simulink model "dynamics_working_version_02_12"  (R2019a)
settings: Solver=FixedStepAuto  StartTime=0.0  StopTime=10.0  FixedStep=3.90625e-3  RelTol=1e-3
values from neighbouring files (symbols this model uses):
  b = 0.033    [set_params.m]
  g = 9.81    [set_params.m]
  I_CF_1 = [16.823890  -1.224320  -0.716891 ... (first row only)    [set_params.m]
  I_CF_1_inv = inv(I_CF_1)    [set_params.m]
  I_rzz = 9.3e-6    (= 9.3e-06)    [set_params.m]
  k_f = 1.6e-4    (= 0.00016)    [set_params.m]
  k_m = 1e-8    (= 1e-08)    [set_params.m]
  kx = 10.25e-4    (= 0.001025)    [set_params.m]
  ky = 10.25e-4    (= 0.001025)    [set_params.m]
  kz = 7.553e-4    (= 0.0007553)    [set_params.m]
  l = 0.033    [set_params.m]
  m_CF = 0.028    [set_params.m]
  omega_n = 50    [set_params.m]
  T = 1/15    (= 0.0666666666667)    [inner_pd.m]    (also in inner_pd_cs.m; outer_pd.m; outer_pd_cs.m; set_params.m)
  zeta = 0.55    [set_params.m]
libraries: sharedutil x2, simulink x1
settings Model: Creator=evgheniivolodscoi  LastModifiedBy=evgheniivolodscoi

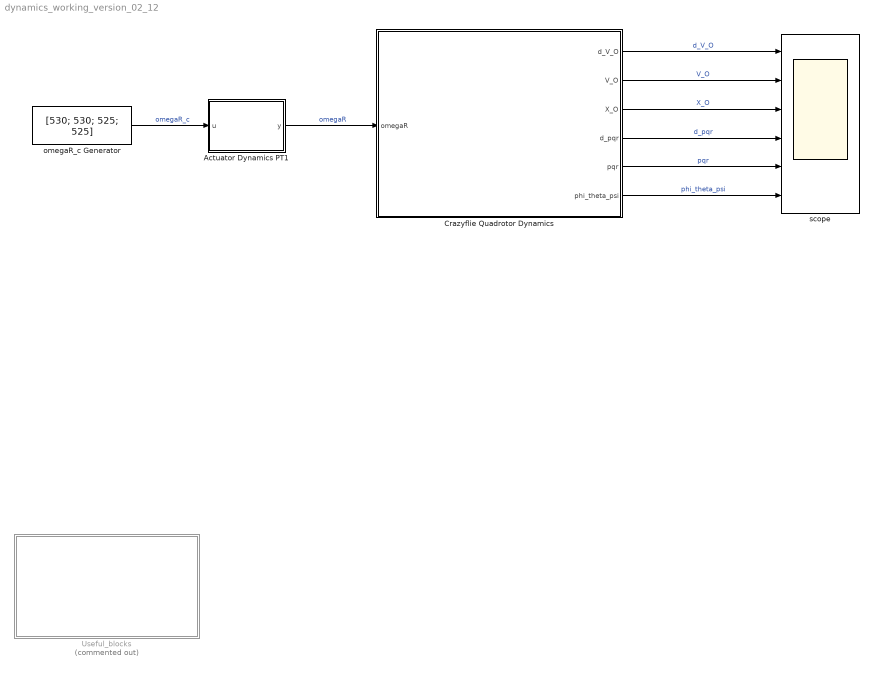
== system dynamics_working_version_02_12 ==
  Actuator Dynamics PT1 : Subsystem
  Crazyflie Quadrotor Dynamics : Subsystem
  "Useful_blocks " : Subsystem  Commented=on
  "omegaR_c Generator " : Constant  Value=[530; 530; 525; 525]
  scope : Scope  NumInputPorts=6
  wires:
  Crazyflie Quadrotor Dynamics/6(phi_theta_psi) -> scope/6  "phi_theta_psi"
  Actuator Dynamics PT1/1(y) -> Crazyflie Quadrotor Dynamics/1(omegaR)  "omegaR"
  Crazyflie Quadrotor Dynamics/4(d_pqr) -> scope/4  "d_pqr"
  Crazyflie Quadrotor Dynamics/3(X_O) -> scope/3  "X_O"
  Crazyflie Quadrotor Dynamics/2(V_O) -> scope/2  "V_O"
  Crazyflie Quadrotor Dynamics/1(d_V_O) -> scope/1  "d_V_O"
  "omegaR_c Generator "/1 -> Actuator Dynamics PT1/1(u)  "omegaR_c"
  Crazyflie Quadrotor Dynamics/5(pqr) -> scope/5  "pqr"

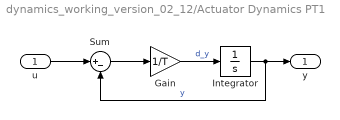
== system dynamics_working_version_02_12/Actuator Dynamics PT1 ==
  u : Inport
  Gain : Gain  Gain=1/T
  Integrator : Integrator
  Sum : Sum  Inputs=|+-
  y : Outport
  wires:
  Integrator/1 -> Sum/2, y/1  "y"
  u/1 -> Sum/1
  Gain/1 -> Integrator/1  "d_y"
  Sum/1 -> Gain/1

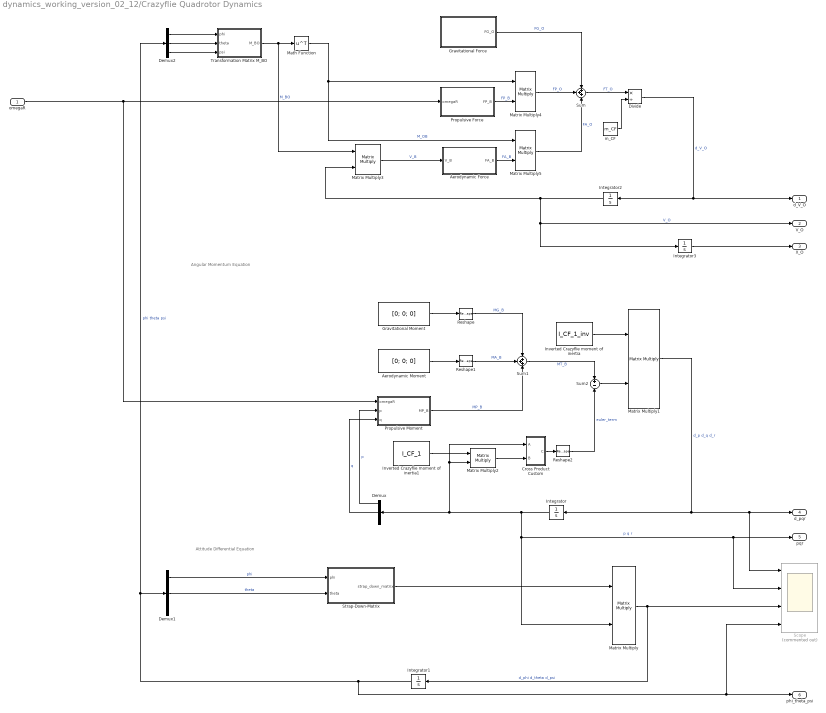
== system dynamics_working_version_02_12/Crazyflie Quadrotor Dynamics ==
  note: Angular Momentum Equation
  note: Attitude Differential Equation
  omegaR : Inport
  Aerodynamic Force : Subsystem
  Aerodynamic Moment : Constant  Value=[0; 0; 0]
  Cross Product Custom : Subsystem
  Demux : Demux  Outputs=3
  Demux1 : Demux  Outputs=3
  Demux2 : Demux  Outputs=3
  Divide : Product  Inputs=*/
  "Gravitational Force " : Subsystem
  Gravitational Moment : Constant  Value=[0; 0; 0]
  Integrator{,1..3} (4 alike) : Integrator  InitialCondition=[0; 0; 0]
  Inverted Crazyflie moment of inertia : Constant  Value=I_CF_1_inv
  Inverted Crazyflie moment of inertia1 : Constant  Value=I_CF_1
  Math Function : Math  Operator=transpose  SaturateOnIntegerOverflow=on
  Matrix Multiply{,1..5} (6 alike) : Product  Multiplication=Matrix(*)
  Propulsive Force : Subsystem
  Propulsive Moment : Subsystem
  Reshape : Reshape  OutputDimensionality=Column vector (2-D)
  Reshape1 : Reshape  OutputDimensionality=Column vector (2-D)
  Reshape2 : Reshape  OutputDimensionality=Column vector (2-D)
  Scope : Scope  Commented=on  NumInputPorts=4
  Strap-Down-Matrix : Subsystem
  Sum : Sum  Inputs=+++
  Sum1 : Sum  Inputs=+++
  Sum2 : Sum  Inputs=+-
  Transformation Matrix M_BO : Subsystem
  m_CF : Constant  Value=m_CF
  d_V_O : Outport
  V_O : Outport  Port=2
  X_O : Outport  Port=3
  d_pqr : Outport  Port=4
  pqr : Outport  Port=5
  phi_theta_psi : Outport  Port=6
  wires:
  Aerodynamic Moment/1 -> Reshape1/1
  Matrix Multiply1/1 -> Integrator/1, Scope/1, d_pqr/1  "d_p d_q d_r"
  Demux1/2 -> Strap-Down-Matrix/2(theta)  "theta"
  Inverted Crazyflie moment of inertia/1 -> Matrix Multiply1/1
  Integrator1/1 -> Demux2/1, Demux1/1, Scope/4, phi_theta_psi/1  "phi theta psi"
  Demux/1 -> Propulsive Moment/2(p)  "p"
  Integrator/1 -> Demux/1, Cross Product Custom/1(A), Matrix Multiply2/2, Matrix Multiply/2, Scope/2, pqr/1  "p q r"
  Propulsive Force/1(FP_B) -> Matrix Multiply4/2  "FP_B"
  "Gravitational Force "/1(FG_O) -> Sum/1  "FG_O"
  Matrix Multiply4/1 -> Sum/2  "FP_O"
  Propulsive Moment/1(MP_B) -> Sum1/3  "MP_B"
  Sum/1 -> Divide/1  "FT_O"
  Demux2/2 -> Transformation Matrix M_BO/2(theta)
  m_CF/1 -> Divide/2
  Gravitational Moment/1 -> Reshape/1
  Transformation Matrix M_BO/1(M_BO) -> Matrix Multiply3/1, Math Function/1  "M_BO"
  Aerodynamic Force/1(FA_B) -> Matrix Multiply5/2  "FA_B"
  Matrix Multiply2/1 -> Cross Product Custom/2(B)
  Cross Product Custom/1(C) -> Reshape2/1
  Matrix Multiply/1 -> Integrator1/1, Scope/3  "d_phi d_theta d_psi"
  Matrix Multiply3/1 -> Aerodynamic Force/1(V_B)  "V_B"
  Demux2/1 -> Transformation Matrix M_BO/1(phi)
  Math Function/1 -> Matrix Multiply4/1, Matrix Multiply5/1  "M_OB"
  Matrix Multiply5/1 -> Sum/3  "FA_O"
  Strap-Down-Matrix/1(strap_down_matrix) -> Matrix Multiply/1
  Demux2/3 -> Transformation Matrix M_BO/3(psi)
  Demux1/1 -> Strap-Down-Matrix/1(phi)  "phi"
  Sum1/1 -> Sum2/1  "MT_B"
  Demux/2 -> Propulsive Moment/3(q)  "q"
  Reshape/1 -> Sum1/1  "MG_B"
  Reshape1/1 -> Sum1/2  "MA_B"
  Reshape2/1 -> Sum2/2  "euler_term"
  omegaR/1 -> Propulsive Moment/1(omegaR), Propulsive Force/1(omegaR)
  Divide/1 -> d_V_O/1, Integrator2/1  "d_V_O"
  Integrator2/1 -> Integrator3/1, V_O/1, Matrix Multiply3/2  "V_O"
  Integrator3/1 -> X_O/1
  Sum2/1 -> Matrix Multiply1/2
  Inverted Crazyflie moment of inertia1/1 -> Matrix Multiply2/1

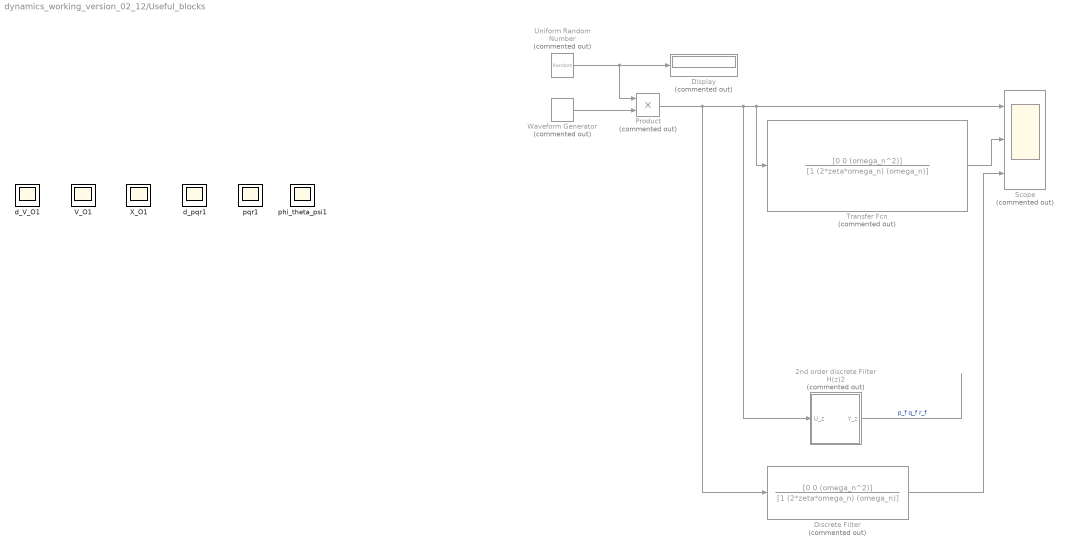
== system dynamics_working_version_02_12/Useful_blocks  ==
  2nd order discrete Filter H(z)2 : Subsystem  Commented=on
  Discrete Filter : DiscreteFilter  Commented=on  Numerator=[0 0 (omega_n^2)]  Denominator=[1 (2*zeta*omega_n) (omega_n)]
  Display : Display  Commented=on
  Product : Product  Commented=on
  Scope : Scope  Commented=on  NumInputPorts=3
  Transfer Fcn : TransferFcn  Commented=on  Numerator=[0 0 (omega_n^2)]  Denominator=[1 (2*zeta*omega_n) (omega_n)]
  Uniform Random Number : UniformRandomNumber  Commented=on  SampleTime=0.1
  V_O1 : Scope
  Waveform Generator : simulink/Sources/Waveform Generator  Commented=on  OutMin=[]  OutMax=[]  OutDataTypeStr=double  SelectedSignal=1  Signals=sin('Amplitude', 2, 'Frequency', 5, 'Phase', 0)  BlockNames=MultiportSwitch_c57f81d41abc4d6  SampleTime=0.1
      settings: SourceProductName=Simulink
  X_O1 : Scope
  d_V_O1 : Scope
  d_pqr1 : Scope
  phi_theta_psi1 : Scope
  pqr1 : Scope
  wires:
  ? -> pqr1/1
  ? -> d_V_O1/1
  ? -> V_O1/1
  ? -> phi_theta_psi1/1
  ? -> X_O1/1
  ? -> d_pqr1/1
  Product/1 -> Discrete Filter/1, 2nd order discrete Filter H(z)2/1(U_z), Transfer Fcn/1, Scope/1
  Discrete Filter/1 -> Scope/3
  2nd order discrete Filter H(z)2/1(Y_z) -> ?  "p_f q_f r_f"
  Waveform Generator/1 -> Product/2
  Transfer Fcn/1 -> Scope/2
  Uniform Random Number/1 -> Product/1, Display/1

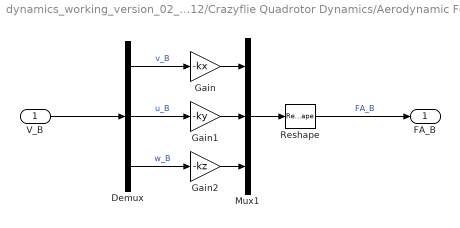
== system dynamics_working_version_02_12/Crazyflie Quadrotor Dynamics/Aerodynamic Force ==
  V_B : Inport
  Demux : Demux  Outputs=3
  Gain : Gain  Gain=-kx
  Gain1 : Gain  Gain=-ky
  Gain2 : Gain  Gain=-kz
  Mux1 : Mux  Inputs=3
  Reshape : Reshape  OutputDimensionality=Column vector (2-D)
  FA_B : Outport
  wires:
  Gain2/1 -> Mux1/3
  Mux1/1 -> Reshape/1
  Gain1/1 -> Mux1/2
  Gain/1 -> Mux1/1
  Demux/2 -> Gain1/1  "u_B"
  V_B/1 -> Demux/1
  Demux/3 -> Gain2/1  "w_B"
  Demux/1 -> Gain/1  "v_B"
  Reshape/1 -> FA_B/1  "FA_B"

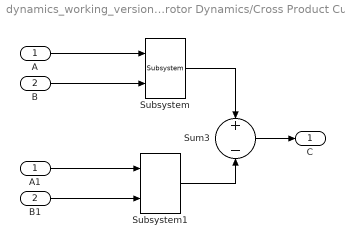
== system dynamics_working_version_02_12/Crazyflie Quadrotor Dynamics/Cross Product Custom ==
  A : Inport
  B : Inport  Port=2
  A1 : InportShadow
  B1 : InportShadow  Port=2
  Subsystem : sharedutil/3x3 Cross Product/Subsystem  SystemSampleTime=-1
      settings: SourceProductName=Aerospace Blockset  SourceProductBaseCode=AE
  Subsystem1 : sharedutil/3x3 Cross Product/Subsystem1  SystemSampleTime=-1
      settings: SourceProductName=Aerospace Blockset  SourceProductBaseCode=AE
  Sum3 : Sum  Inputs=+|-  SaturateOnIntegerOverflow=on  InputSameDT=on  OutDataTypeStr=Inherit: Same as first input
  C : Outport
  wires:
  A1/1 -> Subsystem1/1
  A/1 -> Subsystem/1
  Subsystem1/1 -> Sum3/2
  B/1 -> Subsystem/2
  Sum3/1 -> C/1
  B1/1 -> Subsystem1/2
  Subsystem/1 -> Sum3/1

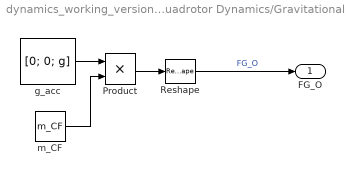
== system dynamics_working_version_02_12/Crazyflie Quadrotor Dynamics/Gravitational Force  ==
  Product : Product
  Reshape : Reshape  OutputDimensionality=Column vector (2-D)
  g_acc : Constant  Value=[0; 0; g]
  m_CF : Constant  Value=m_CF
  FG_O : Outport
  wires:
  m_CF/1 -> Product/2
  g_acc/1 -> Product/1
  Product/1 -> Reshape/1
  Reshape/1 -> FG_O/1  "FG_O"

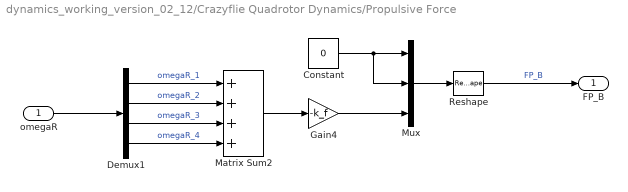
== system dynamics_working_version_02_12/Crazyflie Quadrotor Dynamics/Propulsive Force ==
  omegaR : Inport
  Constant : Constant  Value=0
  Demux1 : Demux
  Gain4 : Gain  Gain=-k_f
  Matrix Sum2 : Sum  Inputs=++++
  Mux : Mux  Inputs=3
  Reshape : Reshape  OutputDimensionality=Column vector (2-D)
  FP_B : Outport
  wires:
  Gain4/1 -> Mux/3
  Demux1/2 -> Matrix Sum2/2  "omegaR_2"
  omegaR/1 -> Demux1/1
  Matrix Sum2/1 -> Gain4/1
  Mux/1 -> Reshape/1
  Demux1/4 -> Matrix Sum2/4  "omegaR_4"
  Demux1/1 -> Matrix Sum2/1  "omegaR_1"
  Demux1/3 -> Matrix Sum2/3  "omegaR_3"
  Reshape/1 -> FP_B/1  "FP_B"
  Constant/1 -> Mux/2, Mux/1

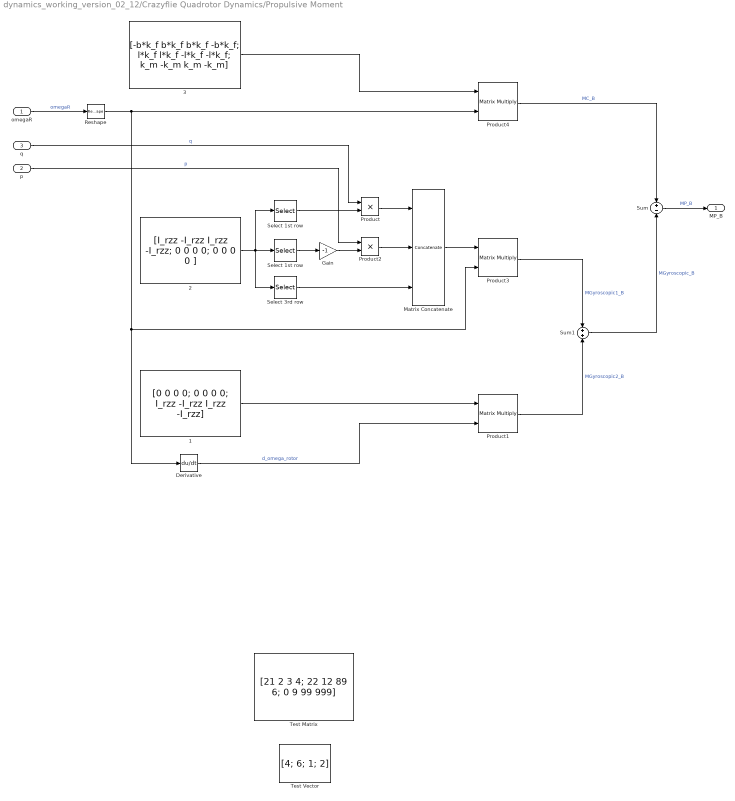
== system dynamics_working_version_02_12/Crazyflie Quadrotor Dynamics/Propulsive Moment ==
  omegaR : Inport
  p : Inport  Port=2
  q : Inport  Port=3
  "  1" : Constant  Value=[0 0 0 0; 0 0 0 0; I_rzz -I_rzz I_rzz -I_rzz]
  "  2" : Constant  Value=[I_rzz -I_rzz I_rzz -I_rzz; 0 0 0 0; 0 0 0 0 ]
  "  3" : Constant  Value=[-b*k_f b*k_f b*k_f -b*k_f; l*k_f l*k_f -l*k_f -l*k_f; k_m -k_m k_m -k_m]
  "  Test Matrix" : Constant  Value=[21 2 3 4; 22 12 89 6; 0 9 99 999]
  Derivative : Derivative
  Gain : Gain  Gain=-1
  Matrix Concatenate : Concatenate  NumInputs=3  Mode=Multidimensional array
  Product : Product
  Product1 : Product  Multiplication=Matrix(*)
  Product2 : Product
  Product3 : Product  Multiplication=Matrix(*)
  Product4 : Product  Multiplication=Matrix(*)
  Reshape : Reshape  OutputDimensionality=Column vector (2-D)
  Select 1st row : Selector  NumberOfDimensions=2  InputPortWidth=3  IndexOptions=Index vector (dialog),Index vector (dialog)  Indices=[1],1:4  OutputSizes=1,1
  "Select 1st row " : Selector  NumberOfDimensions=2  InputPortWidth=3  IndexOptions=Index vector (dialog),Index vector (dialog)  Indices=[1],1:4  OutputSizes=1,1
  Select 3rd row : Selector  NumberOfDimensions=2  InputPortWidth=3  IndexOptions=Index vector (dialog),Index vector (dialog)  Indices=3,1:4  OutputSizes=1,1
  Sum : Sum  Inputs=+-
  Sum1 : Sum
  Test Vector : Constant  Value=[4; 6; 1; 2]
  MP_B : Outport
  wires:
  omegaR/1 -> Reshape/1  "omegaR"
  Product4/1 -> Sum/1  "MC_B"
  Sum/1 -> MP_B/1  "MP_B"
  Sum1/1 -> Sum/2  "MGyroscopic_B"
  "Select 1st row "/1 -> Gain/1
  "  2"/1 -> Select 1st row/1, Select 3rd row/1, "Select 1st row "/1
  Select 1st row/1 -> Product/2
  Product/1 -> Matrix Concatenate/1
  Product2/1 -> Matrix Concatenate/2
  Select 3rd row/1 -> Matrix Concatenate/3
  p/1 -> Product2/1  "p"
  Product3/1 -> Sum1/1  "MGyroscopic1_B"
  "  1"/1 -> Product1/1
  Derivative/1 -> Product1/2  "d_omega_rotor"
  Product1/1 -> Sum1/2  "MGyroscopic2_B"
  Gain/1 -> Product2/2
  q/1 -> Product/1  "q"
  Reshape/1 -> Product4/2, Derivative/1, Product3/2
  "  3"/1 -> Product4/1
  Matrix Concatenate/1 -> Product3/1

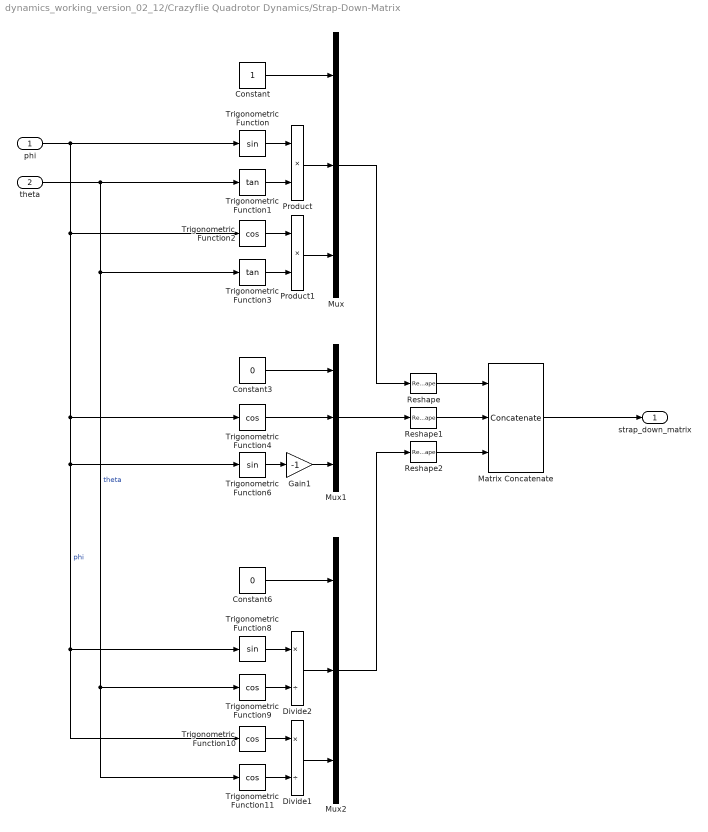
== system dynamics_working_version_02_12/Crazyflie Quadrotor Dynamics/Strap-Down-Matrix ==
  phi : Inport
  theta : Inport  Port=2
  Constant : Constant
  Constant3 : Constant  Value=0
  Constant6 : Constant  Value=0
  Divide1 : Product  Inputs=*/
  Divide2 : Product  Inputs=*/
  Gain1 : Gain  Gain=-1
  Matrix Concatenate : Concatenate  NumInputs=3  Mode=Multidimensional array
  Mux : Mux  Inputs=3
  Mux1 : Mux  Inputs=3
  Mux2 : Mux  Inputs=3
  Product : Product
  Product1 : Product
  Reshape : Reshape  OutputDimensionality=Row vector (2-D)
  Reshape1 : Reshape  OutputDimensionality=Row vector (2-D)
  Reshape2 : Reshape  OutputDimensionality=Row vector (2-D)
  Trigonometric Function : Trigonometry
  Trigonometric Function1 : Trigonometry  Operator=tan
  Trigonometric Function{2,4,9..11} (5 alike) : Trigonometry  Operator=cos
  Trigonometric Function3 : Trigonometry  Operator=tan
  Trigonometric Function6 : Trigonometry
  Trigonometric Function8 : Trigonometry
  strap_down_matrix : Outport
  wires:
  phi/1 -> Trigonometric Function/1, Trigonometric Function2/1, Trigonometric Function4/1, Trigonometric Function6/1, Trigonometric Function8/1, Trigonometric Function10/1  "phi"
  Constant/1 -> Mux/1
  Divide2/1 -> Mux2/2
  Trigonometric Function11/1 -> Divide1/2
  Trigonometric Function10/1 -> Divide1/1
  Mux1/1 -> Reshape1/1
  Trigonometric Function1/1 -> Product/2
  Trigonometric Function8/1 -> Divide2/1
  Mux2/1 -> Reshape2/1
  Trigonometric Function6/1 -> Gain1/1
  Trigonometric Function9/1 -> Divide2/2
  Divide1/1 -> Mux2/3
  Product/1 -> Mux/2
  Trigonometric Function2/1 -> Product1/1
  Trigonometric Function3/1 -> Product1/2
  theta/1 -> Trigonometric Function1/1, Trigonometric Function9/1, Trigonometric Function11/1, Trigonometric Function3/1  "theta"
  Reshape2/1 -> Matrix Concatenate/3
  Trigonometric Function/1 -> Product/1
  Trigonometric Function4/1 -> Mux1/2
  Constant3/1 -> Mux1/1
  Reshape/1 -> Matrix Concatenate/1
  Constant6/1 -> Mux2/1
  Reshape1/1 -> Matrix Concatenate/2
  Product1/1 -> Mux/3
  Mux/1 -> Reshape/1
  Matrix Concatenate/1 -> strap_down_matrix/1
  Gain1/1 -> Mux1/3

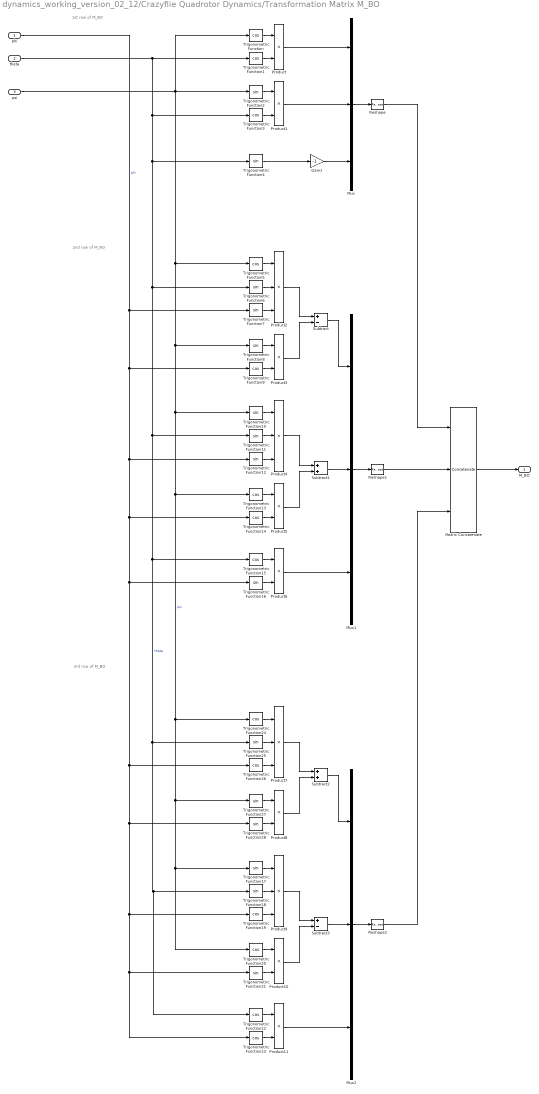
== system dynamics_working_version_02_12/Crazyflie Quadrotor Dynamics/Transformation Matrix M_BO ==
  note: 1st row of M_BO
  note: 2nd row of M_BO
  note: 3rd row of M_BO
  phi : Inport
  theta : Inport  Port=2
  psi : Inport  Port=3
  Gain1 : Gain  Gain=-1
  Matrix Concatenate : Concatenate  NumInputs=3  Mode=Multidimensional array
  Mux : Mux  Inputs=3
  Mux1 : Mux  Inputs=3
  Mux2 : Mux  Inputs=3
  Product{,1,3,5..6,8,10..11} (8 alike) : Product
  Product{2,4,7,9} (4 alike) : Product  Inputs=3
  Reshape : Reshape  OutputDimensionality=Row vector (2-D)
  Reshape1 : Reshape  OutputDimensionality=Row vector (2-D)
  Reshape2 : Reshape  OutputDimensionality=Row vector (2-D)
  Subtract : Sum  Inputs=+-
  Subtract1 : Sum
  Subtract2 : Sum
  Subtract3 : Sum  Inputs=+-
  Trigonometric Function{,1,3,5,9,13..15,19..20,22..24,26} (14 alike) : Trigonometry  Operator=cos
  Trigonometric Function{2,4,6..8,10..12,16..18,21,25,27..28} (15 alike) : Trigonometry
  M_BO : Outport
  wires:
  Matrix Concatenate/1 -> M_BO/1
  Trigonometric Function24/1 -> Product7/1
  Trigonometric Function25/1 -> Product7/2
  Trigonometric Function26/1 -> Product7/3
  Trigonometric Function27/1 -> Product8/1
  Trigonometric Function28/1 -> Product8/2
  Product7/1 -> Subtract2/1
  Product8/1 -> Subtract2/2
  Product10/1 -> Subtract3/2
  Product9/1 -> Subtract3/1
  Trigonometric Function21/1 -> Product10/2
  Trigonometric Function20/1 -> Product10/1
  Trigonometric Function19/1 -> Product9/3
  Trigonometric Function18/1 -> Product9/2
  Trigonometric Function17/1 -> Product9/1
  Trigonometric Function23/1 -> Product11/2
  Trigonometric Function22/1 -> Product11/1
  Subtract2/1 -> Mux2/1
  Product11/1 -> Mux2/3
  Subtract3/1 -> Mux2/2
  Mux2/1 -> Reshape2/1
  Reshape2/1 -> Matrix Concatenate/3
  Reshape1/1 -> Matrix Concatenate/2
  Mux1/1 -> Reshape1/1
  Subtract1/1 -> Mux1/2
  Product6/1 -> Mux1/3
  Subtract/1 -> Mux1/1
  Trigonometric Function15/1 -> Product6/1
  Trigonometric Function16/1 -> Product6/2
  Trigonometric Function10/1 -> Product4/1
  Trigonometric Function11/1 -> Product4/2
  Trigonometric Function12/1 -> Product4/3
  Trigonometric Function13/1 -> Product5/1
  Trigonometric Function14/1 -> Product5/2
  Product4/1 -> Subtract1/1
  Product5/1 -> Subtract1/2
  Product3/1 -> Subtract/2
  Product2/1 -> Subtract/1
  Trigonometric Function9/1 -> Product3/2
  Trigonometric Function8/1 -> Product3/1
  phi/1 -> Trigonometric Function7/1, Trigonometric Function9/1, Trigonometric Function12/1, Trigonometric Function14/1, Trigonometric Function16/1, Trigonometric Function26/1, Trigonometric Function28/1, Trigonometric Function19/1, Trigonometric Function21/1, Trigonometric Function23/1  "phi"
  Trigonometric Function7/1 -> Product2/3
  theta/1 -> Trigonometric Function1/1, Trigonometric Function3/1, Trigonometric Function4/1, Trigonometric Function6/1, Trigonometric Function11/1, Trigonometric Function15/1, Trigonometric Function25/1, Trigonometric Function18/1, Trigonometric Function22/1  "theta"
  Trigonometric Function6/1 -> Product2/2
  Trigonometric Function5/1 -> Product2/1
  Reshape/1 -> Matrix Concatenate/1
  Mux/1 -> Reshape/1
  Trigonometric Function4/1 -> Gain1/1
  Product1/1 -> Mux/2
  Product/1 -> Mux/1
  Trigonometric Function2/1 -> Product1/1
  Trigonometric Function3/1 -> Product1/2
  psi/1 -> Trigonometric Function2/1, Trigonometric Function/1, Trigonometric Function5/1, Trigonometric Function8/1, Trigonometric Function10/1, Trigonometric Function13/1, Trigonometric Function24/1, Trigonometric Function27/1, Trigonometric Function17/1, Trigonometric Function20/1  "psi"
  Trigonometric Function1/1 -> Product/2
  Trigonometric Function/1 -> Product/1
  Gain1/1 -> Mux/3

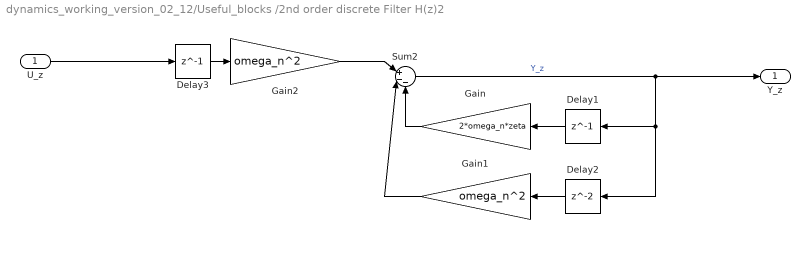
== system dynamics_working_version_02_12/Useful_blocks /2nd order discrete Filter H(z)2 ==
  U_z : Inport
  Delay1 : Delay  DelayLength=1  InitialCondition=0
  Delay2 : Delay  InitialCondition=0
  Delay3 : Delay  DelayLength=1  InitialCondition=0
  Gain : Gain  Gain=2*omega_n*zeta
  Gain1 : Gain  Gain=omega_n^2
  Gain2 : Gain  Gain=omega_n^2
  Sum2 : Sum  Inputs=|+--
  Y_z : Outport
  wires:
  Gain/1 -> Sum2/3
  U_z/1 -> Delay3/1
  Delay1/1 -> Gain/1
  Delay2/1 -> Gain1/1
  Gain1/1 -> Sum2/2
  Delay3/1 -> Gain2/1
  Gain2/1 -> Sum2/1
  Sum2/1 -> Y_z/1, Delay1/1, Delay2/1  "Y_z"
